simulink model "power_pmmotor"  (Simulink 6.0)
settings: Solver=ode15s  SolverMode=SingleTasking  StartTime=0.0  StopTime=0.06  RelTol=1e-3  AbsTol=1e-3
libraries: powerlib x5
settings Model: Creator=patrice  LastModifiedBy=batserve  ExtModeTrigMode=oneshot  ExtModeArmWhenConnect=off  ExtModeAutoUpdateStatusClock=off
settings DataIOCC: ExternalInput=[]  LimitDataPoints=off  SaveOutput=off  SaveTime=off  SignalLoggingName=sigsOut
settings OptimizationCC: BlockReduction=off  BooleanDataType=off
settings DebuggingCC: CheckExecutionContextPreStartOutputMsg=on  CheckExecutionContextRuntimeOutputMsg=on  SolverPrmCheckMsg=none
settings HardwareCC: TargetUnknown=on
settings RTWCC: TemplateMakefile=grt_unix.tmf

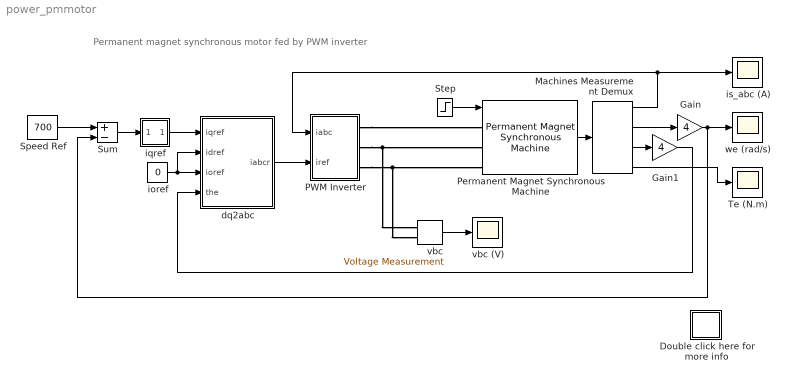
== system power_pmmotor ==
  note: Permanent magnet synchronous motor fed by PWM inverter
  Double click here for more info : Subsystem
      mask Display: disp('?')
  Gain : Gain  Gain=4  SaturateOnIntegerOverflow=on
  Gain1 : Gain  Gain=4  SaturateOnIntegerOverflow=on
  Machines Measurement Demux : powerlib/Machines/Machines Measurement Demux  machType=Permanent magnet synchronous  ssm1=on  ssm2=on  ssm3=on  ssm4=on  ssm5=on  ssm6=on  sm1=on  sm2=on  sm3=on  sm4=on  sm5=on  sm6=on  sm7=on  sm8=on  sm9=on  sm10=on  sm11=on  sm115=off  sm12=off  sm13=off  sm14=off  asm1=on  asm2=on  asm3=on  asm4=on  asm5=on  asm6=on  asm7=on  asm8=on  asm9=on  asm10=on  asm11=on  pmsm1=on  pmsm2=off  pmsm3=off  pmsm4=on  pmsm5=on  pmsm6=on  lastType=4
  PWM Inverter : Subsystem
  Permanent Magnet Synchronous Machine : powerlib/Machines/Permanent Magnet Synchronous Machine  PresetModel=No  ShowDetailedParameters=on  Resistance=2.875  Inductances=[8.5e-3, 8.5e-3]  Flux=0.175  Mechanical="[ 0.8e-3, 0,  4 ]"
      settings: AttributesFormatString=\n
  Speed Ref : Constant  Value=700
  Step : Step  Time=0.04  Before=3  SampleTime=0
  Sum : Sum  Inputs=+-  SaturateOnIntegerOverflow=on  InputSameDT=on
  Te (N.m) : Scope
      settings: TimeRange=0.06  YMin=-20  YMax=35  DataFormat=Structure
  dq2abc : Subsystem
  ioref : Constant  Value=0
  iqref : Subsystem  mask(PI Controller){@1=2.6, @2=50, @3=[-30, 30]}
      mask prompts: @1 "Integral"; @2 "Proportional:"; @3 "Minimum and maximum outputs:"
      mask init:
      | I=@1;P=@2;sat=@3;min=sat(1);max=sat(2);
      mask Display: disp('PI')
  is_abc (A) : Scope
      settings: TimeRange=0.06  YMin=-30  YMax=35  DataFormat=Structure
  vbc : powerlib/Measurements/Voltage Measurement  Tag=PoWeRsYsTeMmEaSuReMeNt  PhasorSimulation=off  OutputType=Magnitude  PSBequivalent=0
  vbc (V) : Scope
      settings: TimeRange=0.06  YMin=-500  YMax=500  DataFormat=Structure
  we (rad/s) : Scope
      settings: TimeRange=0.06  YMin=0  YMax=800  DataFormat=Structure
  wires:
  ioref/1 -> dq2abc/2(idref), dq2abc/3(ioref)
  Sum/1 -> iqref/1(In_1)
  Speed Ref/1 -> Sum/1
  iqref/1(Out_1) -> dq2abc/1(iqref)
  dq2abc/1(iabcr) -> PWM Inverter/2(iref)
  Machines Measurement Demux/1 -> PWM Inverter/1(iabc), is_abc (A)/1
  Machines Measurement Demux/4 -> Te (N.m)/1
  Machines Measurement Demux/2 -> Gain/1
  Gain/1 -> Sum/2, we (rad/s)/1
  Machines Measurement Demux/3 -> Gain1/1
  Gain1/1 -> dq2abc/4(the)
  Step/1 -> Permanent Magnet Synchronous Machine/1
  Permanent Magnet Synchronous Machine/1 -> Machines Measurement Demux/1
  vbc/1 -> vbc (V)/1
  connections:
  PWM Inverter/RConn1 -- Permanent Magnet Synchronous Machine/LConn1
  PWM Inverter/RConn2 -- vbc/LConn1 -- Permanent Magnet Synchronous Machine/LConn2
  PWM Inverter/RConn3 -- Permanent Magnet Synchronous Machine/LConn3 -- vbc/LConn2

== system power_pmmotor/Double click here for more info ==
  note: Observe that the stator currents are quite "noisy," which is to be expected when using PWM inverters. Also, the
      | amplitude of these currents decreases at t = 0.04 s, when the load is decreased. The noise introduced by the PWM
      | inverter is also observed in the electromagnetic torque waveform Te. However, the motor's inertia prevents this
      | noise from appearing in the motor's speed waveform.
  note: A three-phase motor rated 1.1 kW, 220 V, 3000 rpm is fed by a PWM inverter. The PWM inverter is built
      | entirely with standard Simulink blocks. Its output goes through Controlled Voltage Source blocks before
      | being applied to the PMSM block's stator windings. The load torque applied to the  machine's shaft is
      | originally set to its nominal value (3 N.m) and steps down to 1 N.m at t = 0.04 s.
      |
      | Two control loops are used. The inner loop regulates the motor's stator currents. The outer loop controls
      | the motor's speed.
  note: This demonstration illustrates use of the PMSM in a closed-loop
      | speed and current control on a 1.1 kW, 3000 rpm industrial motor
  note: Circuit Description
  note: Demonstration
  note: Louis-A. Dessaint and R. Champagne (Ecole de Technologie Superieure, Montreal)

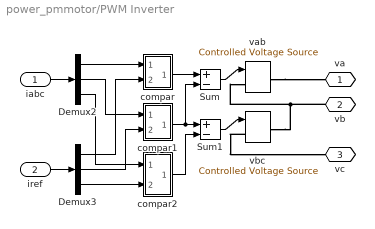
== system power_pmmotor/PWM Inverter ==
  iabc : Inport  Port=1  LatchInput=off
  iref : Inport  Port=2  LatchInput=off
  Demux2 : Demux  Outputs=3
  Demux3 : Demux  Outputs=3
  Sum : Sum  Inputs=+-  SaturateOnIntegerOverflow=on  InputSameDT=on
  Sum1 : Sum  Inputs=+-  SaturateOnIntegerOverflow=on  InputSameDT=on
  compar : Subsystem
  compar1 : Subsystem
  compar2 : Subsystem
  vab : powerlib/Electrical Sources/Controlled Voltage Source  Description=source block  Initialize=on  Amplitude=0  Phase=0  Frequency=0  Measurements=None
      settings: AttributesFormatString=\n
  vbc : powerlib/Electrical Sources/Controlled Voltage Source  Description=source block  Initialize=on  Amplitude=0  Phase=0  Frequency=0  Measurements=None
      settings: AttributesFormatString=\n
  va : PMIOPort  Orientation=left  Port=1  Side=Right
  vb : PMIOPort  Orientation=left  Port=2  Side=Right
  vc : PMIOPort  Orientation=left  Port=3  Side=Right
  wires:
  Demux2/1 -> compar/1(ia)
  Demux2/2 -> compar1/1(ib)
  Demux2/3 -> compar2/1(ic)
  Demux3/3 -> compar2/2(icr)
  Demux3/2 -> compar1/2(ibr)
  Demux3/1 -> compar/2(iar)
  compar/1(va) -> Sum/1
  compar1/1(vb) -> Sum/2, Sum1/1
  compar2/1(vc) -> Sum1/2
  iabc/1 -> Demux2/1
  iref/1 -> Demux3/1
  Sum/1 -> vab/1
  Sum1/1 -> vbc/1
  connections:
  vab/RConn1 -- va/RConn1
  vb/RConn1 -- vab/LConn1 -- vbc/RConn1
  vbc/LConn1 -- vc/RConn1

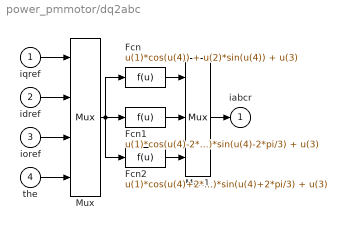
== system power_pmmotor/dq2abc ==
  iqref : Inport  Port=1  LatchInput=off
  idref : Inport  Port=2  LatchInput=off
  ioref : Inport  Port=3  LatchInput=off
  the : Inport  Port=4  LatchInput=off
  Fcn : Fcn  Expr=u(1)*cos(u(4)) + u(2)*sin(u(4)) + u(3)
  Fcn1 : Fcn  Expr=u(1)*cos(u(4)-2*pi/3) + u(2)*sin(u(4)-2*pi/3) + u(3)
  Fcn2 : Fcn  Expr=u(1)*cos(u(4)+2*pi/3) + u(2)*sin(u(4)+2*pi/3) + u(3)
  Mux : Mux
  Mux1 : Mux  Inputs=3
  iabcr : Outport  InitialOutput=0
  wires:
  the/1 -> Mux/4
  ioref/1 -> Mux/3
  idref/1 -> Mux/2
  iqref/1 -> Mux/1
  Mux/1 -> Fcn1/1, Fcn2/1, Fcn/1
  Fcn1/1 -> Mux1/2
  Fcn/1 -> Mux1/1
  Fcn2/1 -> Mux1/3
  Mux1/1 -> iabcr/1

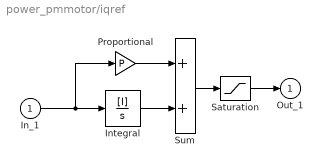
== system power_pmmotor/iqref ==
  In_1 : Inport  Port=1  LatchInput=off
  Integral : TransferFcn  Numerator=[I]  Denominator=[1 0]
  Proportional : Gain  Gain=P  SaturateOnIntegerOverflow=on
  Saturation : Saturate  UpperLimit=max  LowerLimit=min
  Sum : Sum  SaturateOnIntegerOverflow=on  InputSameDT=on
  Out_1 : Outport  InitialOutput=0
  wires:
  Integral/1 -> Sum/2
  In_1/1 -> Integral/1, Proportional/1
  Proportional/1 -> Sum/1
  Sum/1 -> Saturation/1
  Saturation/1 -> Out_1/1

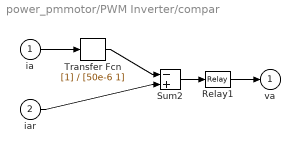
== system power_pmmotor/PWM Inverter/compar ==
  ia : Inport  Port=1  LatchInput=off
  iar : Inport  Port=2  LatchInput=off
  Relay1 : Relay  OnSwitchValue=0.25  OffSwitchValue=-0.25  OnOutputValue=155  OffOutputValue=-155
  Sum2 : Sum  Inputs=-+  SaturateOnIntegerOverflow=on  InputSameDT=on
  Transfer Fcn : TransferFcn  Denominator=[50e-6 1]
  va : Outport  InitialOutput=0
  wires:
  iar/1 -> Sum2/2
  Sum2/1 -> Relay1/1
  Relay1/1 -> va/1
  ia/1 -> Transfer Fcn/1
  Transfer Fcn/1 -> Sum2/1

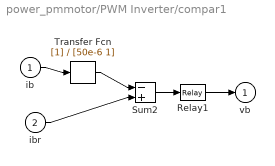
== system power_pmmotor/PWM Inverter/compar1 ==
  ib : Inport  Port=1  LatchInput=off
  ibr : Inport  Port=2  LatchInput=off
  Relay1 : Relay  OnSwitchValue=0.25  OffSwitchValue=-0.25  OnOutputValue=155  OffOutputValue=-155
  Sum2 : Sum  Inputs=-+  SaturateOnIntegerOverflow=on  InputSameDT=on
  Transfer Fcn : TransferFcn  Denominator=[50e-6 1]
  vb : Outport  InitialOutput=0
  wires:
  ibr/1 -> Sum2/2
  Sum2/1 -> Relay1/1
  Relay1/1 -> vb/1
  ib/1 -> Transfer Fcn/1
  Transfer Fcn/1 -> Sum2/1

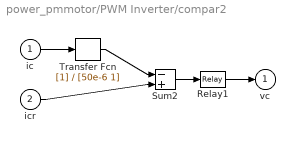
== system power_pmmotor/PWM Inverter/compar2 ==
  ic : Inport  Port=1  LatchInput=off
  icr : Inport  Port=2  LatchInput=off
  Relay1 : Relay  OnSwitchValue=0.25  OffSwitchValue=-0.25  OnOutputValue=155  OffOutputValue=-155
  Sum2 : Sum  Inputs=-+  SaturateOnIntegerOverflow=on  InputSameDT=on
  Transfer Fcn : TransferFcn  Denominator=[50e-6 1]
  vc : Outport  InitialOutput=0
  wires:
  icr/1 -> Sum2/2
  Sum2/1 -> Relay1/1
  Relay1/1 -> vc/1
  ic/1 -> Transfer Fcn/1
  Transfer Fcn/1 -> Sum2/1
